simulink model "PID_auto"  (R2020b)
settings: Solver=VariableStepAuto  StartTime=0.0  StopTime=40  RelTol=1e-3
values from neighbouring files (symbols this model uses):
  Fi = 1/Ti    (= 0.406504065041)    [PID_auto_script.m]
  Kp = 0.6*K_crit    (= 1.266)    [PID_auto_script.m]
  M = 3    [PID_auto_script.m]
  R = 1    [PID_auto_script.m]
  t_switch = 15    [PID_auto_script.m]
  Td = T_estr/8    (= 0.615)    [PID_auto_script.m]
undefined symbols (not defined in the file or in its folder): Kp_a
libraries: cstblocks x4, pid_lib x3, simulink x1
settings Model: Creator=lucas  LastModifiedBy=lucas

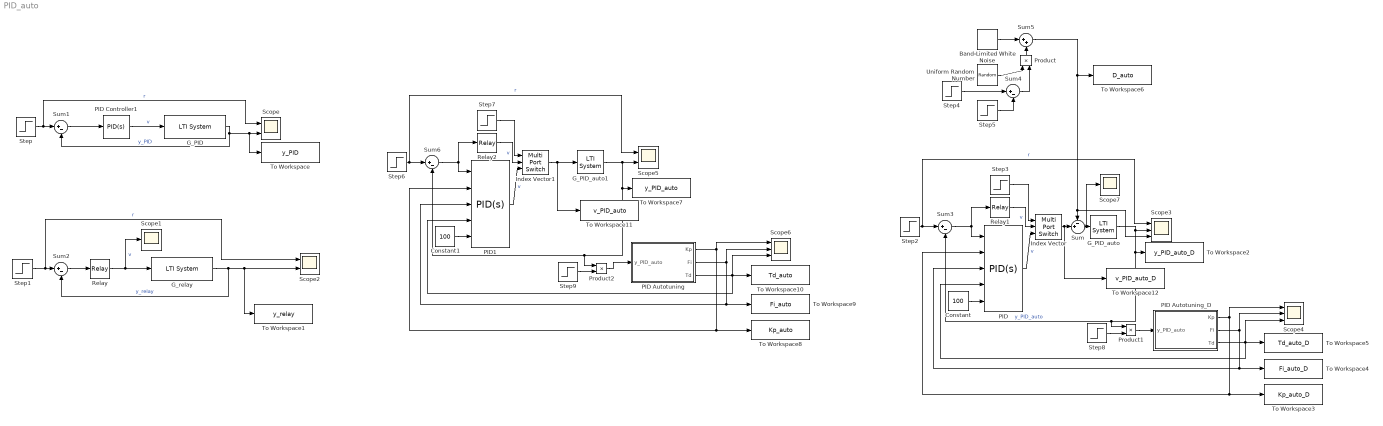
== system PID_auto ==
  Band-Limited White Noise : simulink/Sources/Band-Limited White Noise  Cov=[0.001]  Ts=0.1  seed=[23341]
  Constant : Constant  Value=100
  Constant1 : Constant  Value=100
  G_PID : cstblocks/LTI System  sys=G  IC=[]
  G_PID_auto : cstblocks/LTI System  sys=G  IC=[]
  G_PID_auto1 : cstblocks/LTI System  sys=G  IC=[]
  G_relay : cstblocks/LTI System  sys=G  IC=[]
  Index Vector : MultiPortSwitch  DataPortOrder=Zero-based contiguous  Inputs=2  zeroidx=on
  Index Vector1 : MultiPortSwitch  DataPortOrder=Zero-based contiguous  Inputs=2  zeroidx=on
  PID : pid_lib/PID Controller  Controller=PID  Form=Parallel  TimeDomain=Continuous-time  UseExternalTs=off  SampleTime=-1  IntegratorMethod=Forward Euler  FilterMethod=Forward Euler  ControllerParametersSource=external  P=Kp_a  I=1  D=0  UseFilter=on  N=100  TunerSelectOption=Transfer Function Based (PID Tuner App)  InitialConditionSource=internal  InitialConditionForIntegrator=0  InitialConditionForFilter=0  DifferentiatorICPrevScaledInput=0  ExternalReset=none  TrackingMode=off  Kt=1  LimitOutput=off  SatLimitsSource=internal  UpperSaturationLimit=inf  LowerSaturationLimit=-inf  LinearizeAsGain=on  AntiWindupMode=none  Kb=1  POutMin=[]  POutMax=[]  IOutMin=[]  IOutMax=[]  DOutMin=[]  DOutMax=[]  NOutMin=[]  NOutMax=[]  SumOutMin=[]  SumOutMax=[]  SaturationOutMin=[]  SaturationOutMax=[]  PParamMin=[]  PParamMax=[]  IParamMin=[]  IParamMax=[]  DParamMin=[]  DParamMax=[]  NParamMin=[]  NParamMax=[]  KbParamMin=[]  KbParamMax=[]  KtParamMin=[]  KtParamMax=[]  KbOutMin=[]  KbOutMax=[]  KtOutMin=[]  KtOutMax=[]  IntegratorOutMin=[]  IntegratorOutMax=[]  FilterOutMin=[]  FilterOutMax=[]  SumI1OutMin=[]  SumI1OutMax=[]  SumI2OutMin=[]  SumI2OutMax=[]  SumI3OutMin=[]  SumI3OutMax=[]  SumI4OutMin=[]  SumI4OutMax=[]  SumDOutMin=[]  SumDOutMax=[]  DifferentiatorOutMin=[]  DifferentiatorOutMax=[]  FilterDiffOutCoefMin=[]  FilterDiffOutCoefMax=[]  ReciprocalOutMin=[]  ReciprocalOutMax=[]  SumDenOutMin=[]  SumDenOutMax=[]  SumNumOutMin=[]  SumNumOutMax=[]  DivideOutMin=[]  DivideOutMax=[]  UdiffTsProdOutMin=[]  UdiffTsProdOutMax=[]  NTsProdOutMin=[]  NTsProdOutMax=[]  UintegralTsProdOutMin=[]  UintegralTsProdOutMax=[]  UngainTsProdOutMin=[]  UngainTsProdOutMax=[]  IntegratorContinuousStateAttributes=''  IntegratorStateMustResolveToSignalObject=off  IntegratorRTWStateStorageClass=Auto  FilterContinuousStateAttributes=''  FilterStateMustResolveToSignalObject=off  FilterRTWStateStorageClass=Auto  ParallelPVariant=ExternalParameters  IdealPVariant=Disabled  IVariant=ExternalParameters  DVariant=ExternalParameters  IntegratorVariant=Continuous  SatVariant=Disabled  AWVariant=Passthrough  PCopyVariant=Disabled  TRVariant=Disabled  FdbkBlocksVariant=Forward  IdealPFdbkVariant=Disabled  SatFdbkVariant=Disabled  DerivativeFilterVariant=ContFilter  NVariant=ExternalParameters  NCopyVariant=Disabled  FilterICVariant=InternalICsFilter  IntegratorICVariant=InternalICs  ExternalResetVariant=Disabled  TRSumVariant=Passthrough  SumFdbkVariant=Disabled  SumVariant=Sum_PID  TsampFilterVariant=InternalTs  TsampNgainVariant=Passthrough  TsampIntegralVariant=Passthrough  ExternalSaturationOutDataTypeStr=Inherit: Same as second input
  PID Autotuning : Subsystem
  PID Autotuning_D : Subsystem
  PID Controller1 : pid_lib/PID Controller  Controller=PID  Form=Parallel  TimeDomain=Continuous-time  UseExternalTs=off  SampleTime=-1  IntegratorMethod=Forward Euler  FilterMethod=Forward Euler  ControllerParametersSource=internal  P=Kp  I=Fi  D=Td  UseFilter=on  N=100  TunerSelectOption=Transfer Function Based (PID Tuner App)  InitialConditionSource=internal  InitialConditionForIntegrator=0  InitialConditionForFilter=0  DifferentiatorICPrevScaledInput=0  ExternalReset=none  TrackingMode=off  Kt=1  LimitOutput=off  SatLimitsSource=internal  UpperSaturationLimit=inf  LowerSaturationLimit=-inf  LinearizeAsGain=on  AntiWindupMode=none  Kb=1  POutMin=[]  POutMax=[]  IOutMin=[]  IOutMax=[]  DOutMin=[]  DOutMax=[]  NOutMin=[]  NOutMax=[]  SumOutMin=[]  SumOutMax=[]  SaturationOutMin=[]  SaturationOutMax=[]  PParamMin=[]  PParamMax=[]  IParamMin=[]  IParamMax=[]  DParamMin=[]  DParamMax=[]  NParamMin=[]  NParamMax=[]  KbParamMin=[]  KbParamMax=[]  KtParamMin=[]  KtParamMax=[]  KbOutMin=[]  KbOutMax=[]  KtOutMin=[]  KtOutMax=[]  IntegratorOutMin=[]  IntegratorOutMax=[]  FilterOutMin=[]  FilterOutMax=[]  SumI1OutMin=[]  SumI1OutMax=[]  SumI2OutMin=[]  SumI2OutMax=[]  SumI3OutMin=[]  SumI3OutMax=[]  SumI4OutMin=[]  SumI4OutMax=[]  SumDOutMin=[]  SumDOutMax=[]  DifferentiatorOutMin=[]  DifferentiatorOutMax=[]  FilterDiffOutCoefMin=[]  FilterDiffOutCoefMax=[]  ReciprocalOutMin=[]  ReciprocalOutMax=[]  SumDenOutMin=[]  SumDenOutMax=[]  SumNumOutMin=[]  SumNumOutMax=[]  DivideOutMin=[]  DivideOutMax=[]  UdiffTsProdOutMin=[]  UdiffTsProdOutMax=[]  NTsProdOutMin=[]  NTsProdOutMax=[]  UintegralTsProdOutMin=[]  UintegralTsProdOutMax=[]  UngainTsProdOutMin=[]  UngainTsProdOutMax=[]  IntegratorContinuousStateAttributes=''  IntegratorStateMustResolveToSignalObject=off  IntegratorRTWStateStorageClass=Auto  FilterContinuousStateAttributes=''  FilterStateMustResolveToSignalObject=off  FilterRTWStateStorageClass=Auto  ParallelPVariant=InternalParameters  IdealPVariant=Disabled  IVariant=InternalParameters  DVariant=InternalParameters  IntegratorVariant=Continuous  SatVariant=Disabled  AWVariant=Passthrough  PCopyVariant=Disabled  TRVariant=Disabled  FdbkBlocksVariant=Forward  IdealPFdbkVariant=Disabled  SatFdbkVariant=Disabled  DerivativeFilterVariant=ContFilter  NVariant=InternalParameters  NCopyVariant=Disabled  FilterICVariant=InternalICsFilter  IntegratorICVariant=InternalICs  ExternalResetVariant=Disabled  TRSumVariant=Passthrough  SumFdbkVariant=Disabled  SumVariant=Sum_PID  TsampFilterVariant=InternalTs  TsampNgainVariant=Passthrough  TsampIntegralVariant=Passthrough  ExternalSaturationOutDataTypeStr=Inherit: Same as second input
  PID1 : pid_lib/PID Controller  Controller=PID  Form=Parallel  TimeDomain=Continuous-time  UseExternalTs=off  SampleTime=-1  IntegratorMethod=Forward Euler  FilterMethod=Forward Euler  ControllerParametersSource=external  P=Kp_a  I=1  D=0  UseFilter=on  N=100  TunerSelectOption=Transfer Function Based (PID Tuner App)  InitialConditionSource=internal  InitialConditionForIntegrator=0  InitialConditionForFilter=0  DifferentiatorICPrevScaledInput=0  ExternalReset=none  TrackingMode=off  Kt=1  LimitOutput=off  SatLimitsSource=internal  UpperSaturationLimit=inf  LowerSaturationLimit=-inf  LinearizeAsGain=on  AntiWindupMode=none  Kb=1  POutMin=[]  POutMax=[]  IOutMin=[]  IOutMax=[]  DOutMin=[]  DOutMax=[]  NOutMin=[]  NOutMax=[]  SumOutMin=[]  SumOutMax=[]  SaturationOutMin=[]  SaturationOutMax=[]  PParamMin=[]  PParamMax=[]  IParamMin=[]  IParamMax=[]  DParamMin=[]  DParamMax=[]  NParamMin=[]  NParamMax=[]  KbParamMin=[]  KbParamMax=[]  KtParamMin=[]  KtParamMax=[]  KbOutMin=[]  KbOutMax=[]  KtOutMin=[]  KtOutMax=[]  IntegratorOutMin=[]  IntegratorOutMax=[]  FilterOutMin=[]  FilterOutMax=[]  SumI1OutMin=[]  SumI1OutMax=[]  SumI2OutMin=[]  SumI2OutMax=[]  SumI3OutMin=[]  SumI3OutMax=[]  SumI4OutMin=[]  SumI4OutMax=[]  SumDOutMin=[]  SumDOutMax=[]  DifferentiatorOutMin=[]  DifferentiatorOutMax=[]  FilterDiffOutCoefMin=[]  FilterDiffOutCoefMax=[]  ReciprocalOutMin=[]  ReciprocalOutMax=[]  SumDenOutMin=[]  SumDenOutMax=[]  SumNumOutMin=[]  SumNumOutMax=[]  DivideOutMin=[]  DivideOutMax=[]  UdiffTsProdOutMin=[]  UdiffTsProdOutMax=[]  NTsProdOutMin=[]  NTsProdOutMax=[]  UintegralTsProdOutMin=[]  UintegralTsProdOutMax=[]  UngainTsProdOutMin=[]  UngainTsProdOutMax=[]  IntegratorContinuousStateAttributes=''  IntegratorStateMustResolveToSignalObject=off  IntegratorRTWStateStorageClass=Auto  FilterContinuousStateAttributes=''  FilterStateMustResolveToSignalObject=off  FilterRTWStateStorageClass=Auto  ParallelPVariant=ExternalParameters  IdealPVariant=Disabled  IVariant=ExternalParameters  DVariant=ExternalParameters  IntegratorVariant=Continuous  SatVariant=Disabled  AWVariant=Passthrough  PCopyVariant=Disabled  TRVariant=Disabled  FdbkBlocksVariant=Forward  IdealPFdbkVariant=Disabled  SatFdbkVariant=Disabled  DerivativeFilterVariant=ContFilter  NVariant=ExternalParameters  NCopyVariant=Disabled  FilterICVariant=InternalICsFilter  IntegratorICVariant=InternalICs  ExternalResetVariant=Disabled  TRSumVariant=Passthrough  SumFdbkVariant=Disabled  SumVariant=Sum_PID  TsampFilterVariant=InternalTs  TsampNgainVariant=Passthrough  TsampIntegralVariant=Passthrough  ExternalSaturationOutDataTypeStr=Inherit: Same as second input
  Product : Product
  Product1 : Product
  Product2 : Product
  Relay : Relay  OnSwitchValue=0  OffSwitchValue=0  OnOutputValue=M  OffOutputValue=-M
  Relay1 : Relay  OnSwitchValue=0  OffSwitchValue=0  OnOutputValue=M  OffOutputValue=-M
  Relay2 : Relay  OnSwitchValue=0  OffSwitchValue=0  OnOutputValue=M  OffOutputValue=-M
  Scope : Scope  NumInputPorts=2
  Scope1 : Scope
  Scope2 : Scope  NumInputPorts=2
  Scope3 : Scope  NumInputPorts=3
  Scope4 : Scope  NumInputPorts=3
  Scope5 : Scope  NumInputPorts=2
  Scope6 : Scope  NumInputPorts=3
  Scope7 : Scope
  Step{,1..2,6} (4 alike) : Step  Time=0  After=R  SampleTime=0
  Step3 : Step  Time=25  SampleTime=0
  Step4 : Step  Time=t_switch-5  SampleTime=0
  Step5 : Step  Time=t_switch-4  SampleTime=0
  Step7 : Step  Time=t_switch  SampleTime=0
  Step8 : Step  Time=t_switch  Before=1  After=0  SampleTime=0
  Step9 : Step  Time=t_switch  Before=1  After=0  SampleTime=0
  Sum : Sum  Inputs=-+|
  Sum{1..4,6} (5 alike) : Sum  Inputs=|+-
  Sum5 : Sum  Inputs=|++
  To Workspace : ToWorkspace  VariableName=y_PID  SaveFormat=Timeseries  SampleTime=-1
  To Workspace1 : ToWorkspace  VariableName=y_relay  SaveFormat=Timeseries  SampleTime=-1
  To Workspace10 : ToWorkspace  VariableName=Td_auto  SampleTime=-1
      settings: MaxDataPoints=1  Save2DSignal=2-D array (concatenate along first dimension)
  To Workspace11 : ToWorkspace  VariableName=v_PID_auto  SaveFormat=Timeseries  SampleTime=-1
  To Workspace12 : ToWorkspace  VariableName=v_PID_auto_D  SaveFormat=Timeseries  SampleTime=-1
  To Workspace2 : ToWorkspace  VariableName=y_PID_auto_D  SaveFormat=Timeseries  SampleTime=-1
  To Workspace3 : ToWorkspace  VariableName=Kp_auto_D  SampleTime=-1
      settings: MaxDataPoints=1  Save2DSignal=2-D array (concatenate along first dimension)
  To Workspace4 : ToWorkspace  VariableName=Fi_auto_D  SampleTime=-1
      settings: MaxDataPoints=1  Save2DSignal=2-D array (concatenate along first dimension)
  To Workspace5 : ToWorkspace  VariableName=Td_auto_D  SampleTime=-1
      settings: MaxDataPoints=1  Save2DSignal=2-D array (concatenate along first dimension)
  To Workspace6 : ToWorkspace  VariableName=D_auto  SaveFormat=Timeseries  SampleTime=-1
  To Workspace7 : ToWorkspace  VariableName=y_PID_auto  SaveFormat=Timeseries  SampleTime=-1
  To Workspace8 : ToWorkspace  VariableName=Kp_auto  SampleTime=-1
      settings: MaxDataPoints=1  Save2DSignal=2-D array (concatenate along first dimension)
  To Workspace9 : ToWorkspace  VariableName=Fi_auto  SampleTime=-1
      settings: MaxDataPoints=1  Save2DSignal=2-D array (concatenate along first dimension)
  Uniform Random Number : UniformRandomNumber  Minimum=1  Maximum=2  SampleTime=0.1
  wires:
  Sum1/1 -> PID Controller1/1
  PID Controller1/1 -> G_PID/1  "v"
  G_PID/1 -> To Workspace/1, Scope/2, Sum1/2  "y_PID"
  Step/1 -> Scope/1, Sum1/1  "r"
  G_relay/1 -> Sum2/2, To Workspace1/1, Scope2/2  "y_relay"
  Sum2/1 -> Relay/1
  Relay/1 -> Scope1/1, G_relay/1  "v"
  Step1/1 -> Scope2/1, Sum2/1  "r"
  Sum3/1 -> PID/1, Relay1/1
  G_PID_auto/1 -> Product1/1, Sum3/2, To Workspace2/1, Scope3/2  "y_PID_auto"
  Step2/1 -> Scope3/1, Sum3/1  "r"
  Relay1/1 -> Index Vector/2  "v"
  Step3/1 -> Index Vector/1
  PID Autotuning_D/1(Kp) -> PID/2, To Workspace3/1, Scope4/1
  PID Autotuning_D/2(Fi) -> PID/3, To Workspace4/1, Scope4/2
  PID Autotuning_D/3(Td) -> Scope4/3, PID/4, To Workspace5/1
  PID/1 -> Index Vector/3  "v"
  Constant/1 -> PID/5
  Step5/1 -> Sum4/2
  Sum5/1 -> To Workspace6/1, Scope3/3, Sum/1
  Sum4/1 -> Product/2
  Step4/1 -> Sum4/1
  Product/1 -> Sum5/2
  Uniform Random Number/1 -> Product/1
  Band-Limited White Noise/1 -> Sum5/1
  Relay2/1 -> Index Vector1/2  "v"
  PID1/1 -> Index Vector1/3  "v"
  Step6/1 -> Scope5/1, Sum6/1  "r"
  PID Autotuning/2(Fi) -> PID1/3, To Workspace9/1, Scope6/2
  PID Autotuning/1(Kp) -> PID1/2, To Workspace8/1, Scope6/1
  Step7/1 -> Index Vector1/1
  Constant1/1 -> PID1/5
  Index Vector1/1 -> To Workspace11/1, G_PID_auto1/1
  PID Autotuning/3(Td) -> PID1/4, To Workspace10/1, Scope6/3
  Sum6/1 -> PID1/1, Relay2/1
  Index Vector/1 -> To Workspace12/1, Sum/2
  Sum/1 -> Scope7/1, G_PID_auto/1
  Product1/1 -> PID Autotuning_D/1(y_PID_auto)
  Step8/1 -> Product1/2
  Step9/1 -> Product2/2
  G_PID_auto1/1 -> Sum6/2, Product2/1, To Workspace7/1, Scope5/2
  Product2/1 -> PID Autotuning/1(y_PID_auto)

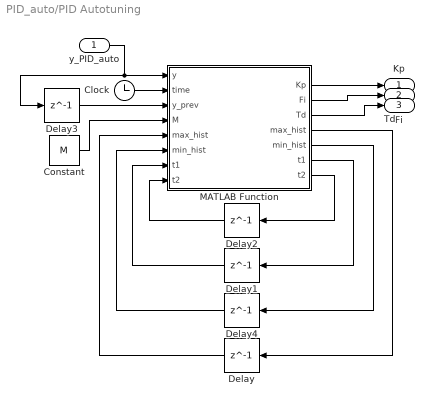
== system PID_auto/PID Autotuning ==
  y_PID_auto : Inport
  Clock : Clock
  Constant : Constant  Value=M
  Delay : Delay  DelayLength=1  InitialCondition=1
  Delay1 : Delay  DelayLength=1  InitialCondition=0
  Delay2 : Delay  DelayLength=1  InitialCondition=1
  Delay3 : Delay  DelayLength=1  InitialCondition=0
  Delay4 : Delay  DelayLength=1  InitialCondition=-1
  MATLAB Function : MATLAB Function  TreatAsAtomicUnit=on
  Kp : Outport
  Fi : Outport  Port=2
  Td : Outport  Port=3
  wires:
  Delay1/1 -> MATLAB Function/7("t1 ")
  MATLAB Function/7(t2) -> Delay2/1
  Constant/1 -> MATLAB Function/4(M)
  MATLAB Function/6(t1) -> Delay1/1
  Delay3/1 -> MATLAB Function/3(y_prev)
  Clock/1 -> MATLAB Function/2(time)
  MATLAB Function/5(min_hist) -> Delay4/1
  y_PID_auto/1 -> Delay3/1, MATLAB Function/1(y)
  MATLAB Function/4(max_hist) -> Delay/1
  Delay2/1 -> MATLAB Function/8("t2 ")
  MATLAB Function/3(Td) -> Td/1
  Delay/1 -> MATLAB Function/5("max_hist ")
  Delay4/1 -> MATLAB Function/6("min_hist ")
  MATLAB Function/2(Fi) -> Fi/1
  MATLAB Function/1(Kp) -> Kp/1

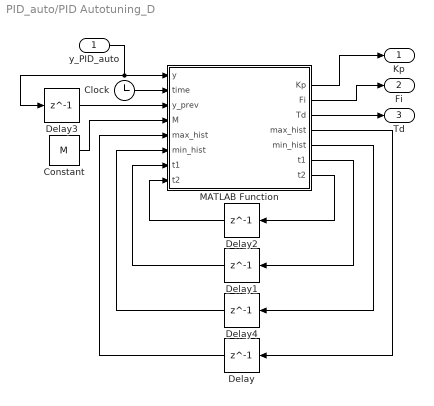
== system PID_auto/PID Autotuning_D ==
  y_PID_auto : Inport
  Clock : Clock
  Constant : Constant  Value=M
  Delay : Delay  DelayLength=1  InitialCondition=1
  Delay1 : Delay  DelayLength=1  InitialCondition=0
  Delay2 : Delay  DelayLength=1  InitialCondition=1
  Delay3 : Delay  DelayLength=1  InitialCondition=0
  Delay4 : Delay  DelayLength=1  InitialCondition=-1
  MATLAB Function : MATLAB Function  TreatAsAtomicUnit=on
  Kp : Outport
  Fi : Outport  Port=2
  Td : Outport  Port=3
  wires:
  Delay1/1 -> MATLAB Function/7("t1 ")
  MATLAB Function/7(t2) -> Delay2/1
  Constant/1 -> MATLAB Function/4(M)
  MATLAB Function/6(t1) -> Delay1/1
  Delay3/1 -> MATLAB Function/3(y_prev)
  Clock/1 -> MATLAB Function/2(time)
  MATLAB Function/5(min_hist) -> Delay4/1
  y_PID_auto/1 -> Delay3/1, MATLAB Function/1(y)
  MATLAB Function/4(max_hist) -> Delay/1
  Delay2/1 -> MATLAB Function/8("t2 ")
  MATLAB Function/3(Td) -> Td/1
  Delay/1 -> MATLAB Function/5("max_hist ")
  Delay4/1 -> MATLAB Function/6("min_hist ")
  MATLAB Function/2(Fi) -> Fi/1
  MATLAB Function/1(Kp) -> Kp/1

== matlab function PID_auto/PID Autotuning/MATLAB Function ==
  data: y input; time input; y_prev input; M input; Kp output; Fi output; Td output; max_hist input; min_hist input; max_hist output; min_hist output; t1 output; t2 output; t1 input; t2 input
function [Kp,Fi,Td,max_hist,min_hist,t1,t2] = autotune_PID(y,time,y_prev,M,max_hist,min_hist,t1,t2)
    if y >= max_hist
        max_hist = y;
    end
    if y <= min_hist
        min_hist = y;
    end
    if y_prev >= max_hist && y <= y_prev && time < 8
        t1 = time-1;
    end
    if y_prev <= min_hist && y >= y_prev && time < 8
        t2 = time-1;
    end
    T_crit = 2*(t2-t1);
    A_crit = (max_hist-min_hist)/2;
    K_crit = 4*M/(pi*A_crit);
    Kp = 0.6*K_crit;
    Ti = T_crit/2;
    Fi = 1/Ti;
    Td = T_crit/8;
end

== matlab function PID_auto/PID Autotuning_D/MATLAB Function ==
  data: y input; time input; y_prev input; M input; Kp output; Fi output; Td output; max_hist input; min_hist input; max_hist output; min_hist output; t1 output; t2 output; t1 input; t2 input
function [Kp,Fi,Td,max_hist,min_hist,t1,t2] = autotune_PID(y,time,y_prev,M,max_hist,min_hist,t1,t2)
    if y >= max_hist
        max_hist = y;
    end
    if y <= min_hist
        min_hist = y;
    end
    if y_prev >= max_hist && y <= y_prev && time < 8
        t1 = time-1;
    end
    if y_prev <= min_hist && y >= y_prev && time < 8
        t2 = time-1;
    end
    T_crit = 2*(t2-t1);
    A_crit = (max_hist-min_hist)/2;
    K_crit = 4*M/(pi*A_crit);
    Kp = 0.6*K_crit;
    Ti = T_crit/2;
    Fi = 1/Ti;
    Td = T_crit/8;
end
